simulink model "kinematicModel"  (R2022b)
settings: Solver=VariableStepAuto  StartTime=0.0  StopTime=10.0  RelTol=1e-3
libraries: roblocks x1
settings Model: Creator=madsm  LastModifiedBy=madsm

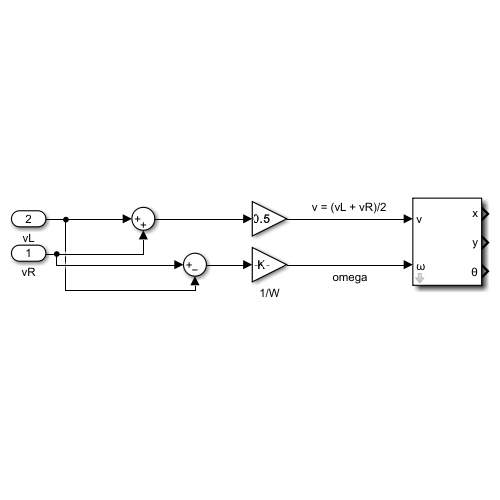
[thumbnail: Simulink's stored preview of the top-level diagram]
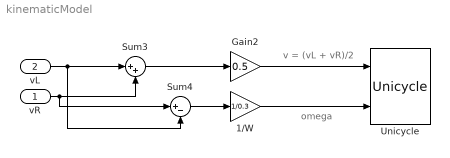
== system kinematicModel ==
  note: omega
  note: v = (vL + vR)/2
  vR : Inport
  vL : Inport  Port=2
  1/W : Gain  Gain=1/0.3
  Gain2 : Gain  Gain=0.5
  Sum3 : Sum  Inputs=|++
  Sum4 : Sum  Inputs=|+-
  Unicycle : roblocks/Vehicles/Unicycle  alim=1  vlim=1  wlim=2  x0=[0, 0, 0]  a=0
  wires:
  vL/1 -> Sum4/2, Sum3/1
  Sum3/1 -> Gain2/1
  vR/1 -> Sum4/1, Sum3/2
  Sum4/1 -> 1/W/1
  1/W/1 -> Unicycle/2
  Gain2/1 -> Unicycle/1
